simulink library "QuaternionLibrary"  (R2015a)
settings: Solver=ode45  StartTime=0.0  StopTime=10.0  RelTol=1e-3
libraries: VectorLibrary x2, ZeroProtectionLibrary x1
settings Model: Creator=Cam  LastModifiedBy=Cam

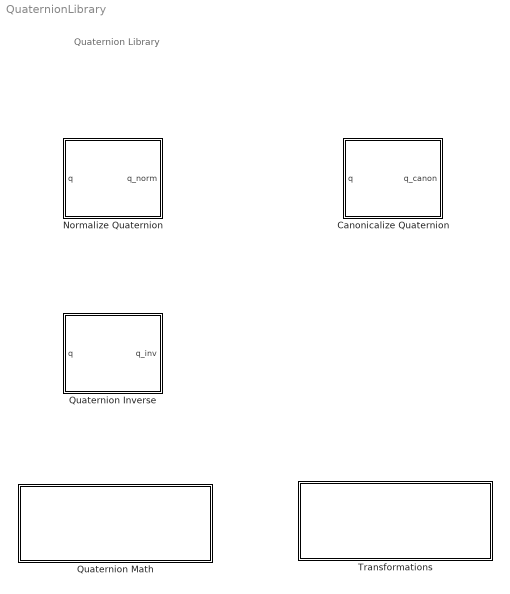
== system QuaternionLibrary ==
  note: Quaternion Library
  Canonicalize Quaternion : Subsystem  mask(Canonicalize Quaternion){}
      mask help: Returns the canonicalized form of the quaternion. This ensures that the angle is less than 180 degrees.
      mask Display: disp('Canonicalize\nQuaternion')
  Normalize Quaternion : Subsystem  mask(Normalize Quaternion){}
      mask help: Normalizes the given quaternion.
      mask Display: disp('Normalize\nQuaternion')
  Quaternion Inverse : Subsystem  mask(Quaternion Inverse){}
      mask help:
      | Returns the inverse of the given quaternion. That is, returns the quaternion that represents a rotation of the same angle, but about the negative of the axis.
      |
      | Exit condition:
      |  - The canonicalization status of the quaternion is preserved.
      mask Display: disp('Quaternion\nInverse')
  Quaternion Math : Subsystem
      mask Display: disp('Quaternion Math')
  Transformations : Subsystem
      mask Display: disp('Transformations')

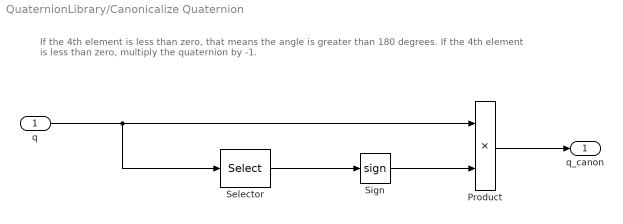
== system QuaternionLibrary/Canonicalize Quaternion ==
  note: If the 4th element is less than zero, that means the angle is greater than 180 degrees.
      | If the 4th element is less than zero, multiply the quaternion by -1.
  q : Inport
  Product : Product
  Selector : Selector  InputPortWidth=4  Indices=[4]
  Sign : Signum
  q_canon : Outport
  wires:
  q/1 -> Selector/1, Product/1
  Product/1 -> q_canon/1
  Sign/1 -> Product/2
  Selector/1 -> Sign/1

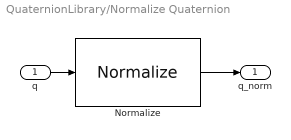
== system QuaternionLibrary/Normalize Quaternion ==
  q : Inport
  Normalize : VectorLibrary/Normalize
  q_norm : Outport
  wires:
  q/1 -> Normalize/1
  Normalize/1 -> q_norm/1

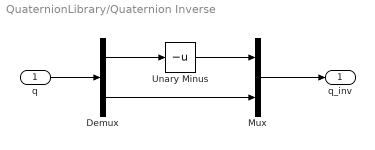
== system QuaternionLibrary/Quaternion Inverse ==
  q : Inport
  Demux : Demux  Outputs=2
  Mux : Mux  Inputs=2
  Unary Minus : UnaryMinus
  q_inv : Outport
  wires:
  Mux/1 -> q_inv/1
  q/1 -> Demux/1
  Demux/1 -> Unary Minus/1
  Unary Minus/1 -> Mux/1
  Demux/2 -> Mux/2

== system QuaternionLibrary/Quaternion Math ==
  note: Quaternion Math

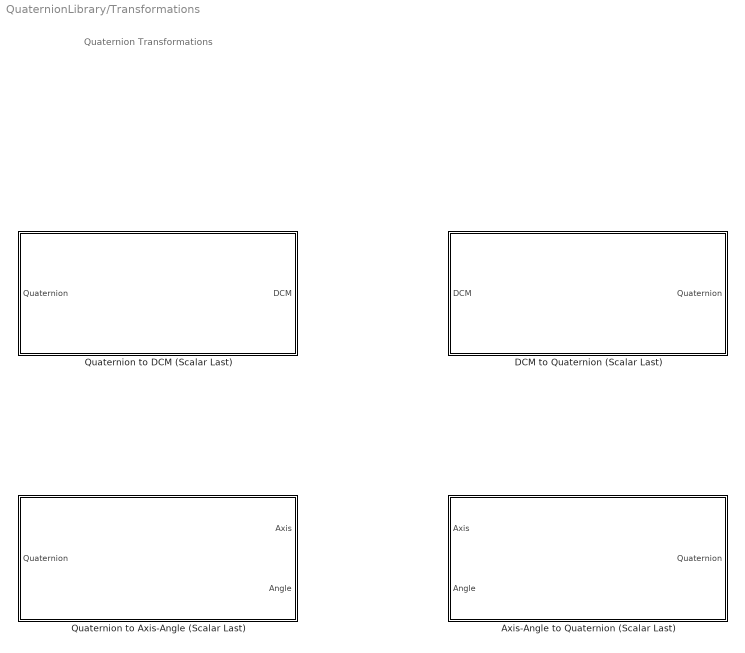
== system QuaternionLibrary/Transformations ==
  note: Quaternion Transformations
  Axis-Angle to Quaternion (Scalar Last) : Subsystem  mask(Axis-Angle to Quaternion){}
      mask help:
      | Returns the quaternion that represents a rotation of the given angle around the given axis.
      |
      | Entry condition:
      |  - Axis vector is normalized.
      mask Display:
      | port_label('input',1,'Axis')
      | port_label('input',2,'Angle')
      | port_label('output',1,'Quaternion')
      | disp('Axis-Angle \nto Quaternion\n')
      | color('red')
      | disp('\n\n(Scalar Last)')
  DCM to Quaternion (Scalar Last) : Subsystem  mask(DCM to Quaternion){}
      mask help:
      | This block transforms a DCM into a Quaternion.
      |
      | Entry condition:
      |  - Rows of DCM must be normalized.
      mask Display:
      | port_label('input',1,'DCM')
      | port_label('output',1,'Quaternion')
      | disp('Quaternion \nto DCM\n')
      | color('red')
      | disp('\n\n(Scalar Last)')
  Quaternion to Axis-Angle (Scalar Last) : Subsystem  mask(Quaternion to Axis-Angle){}
      mask help:
      | Returns the Euler axis and rotation angle about that axis that the quaternion represents.
      |
      | Entry Condition:
      |  - Quaternion is normalized.
      |
      | Exit condition:
      |  - Axis is normalized.
      |  - Canonicalization status is unchanged.
      mask Display:
      | port_label('input',1,'Quaternion')
      | port_label('output',1,'Axis')
      | port_label('output',2,'Angle')
      | disp('Quaternion \nto Axis-Angle\n')
      | color('red')
      | disp('\n\n(Scalar Last)')
  Quaternion to DCM (Scalar Last) : Subsystem  TreatAsAtomicUnit=on  mask(Quaternion to DCM){}
      mask help:
      | This block transforms a Quaternion into a Direction Cosine Matrix.
      |
      | Entry condition:
      |  - Quaternion must be normalized.
      mask Display:
      | port_label('input',1,'Quaternion')
      | port_label('output',1,'DCM')
      | disp('Quaternion \nto DCM\n')
      | color('red')
      | disp('\n\n(Scalar Last)')

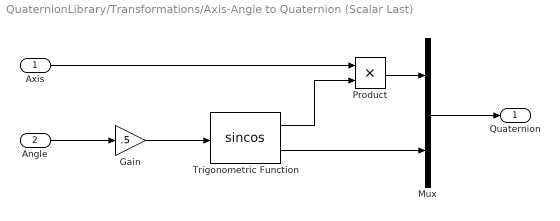
== system QuaternionLibrary/Transformations/Axis-Angle to Quaternion (Scalar Last) ==
  Axis : Inport
  Angle : Inport  Port=2
  Gain : Gain  Gain=.5
  Mux : Mux  Inputs=2
  Product : Product
  Trigonometric Function : Trigonometry  Operator=sincos
  Quaternion : Outport
  wires:
  Mux/1 -> Quaternion/1
  Angle/1 -> Gain/1
  Gain/1 -> Trigonometric Function/1
  Trigonometric Function/2 -> Mux/2
  Axis/1 -> Product/1
  Product/1 -> Mux/1
  Trigonometric Function/1 -> Product/2

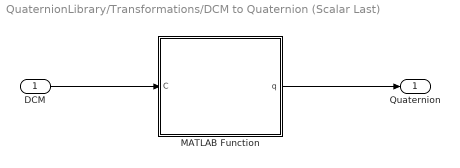
== system QuaternionLibrary/Transformations/DCM to Quaternion (Scalar Last) ==
  DCM : Inport
  MATLAB Function : MATLAB Function  TreatAsAtomicUnit=on
  Quaternion : Outport
  wires:
  DCM/1 -> MATLAB Function/1(C)
  MATLAB Function/1(q) -> Quaternion/1

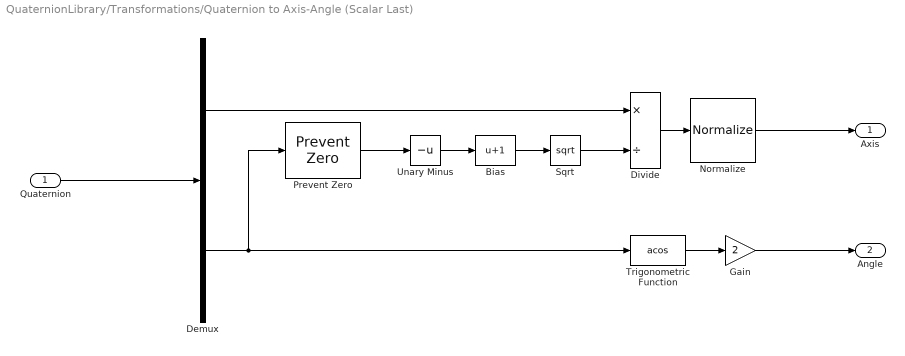
== system QuaternionLibrary/Transformations/Quaternion to Axis-Angle (Scalar Last) ==
  Quaternion : Inport
  Bias : Bias  Bias=1
  Demux : Demux  Outputs=[3 1]
  Divide : Product  Inputs=*/
  Gain : Gain  Gain=2
  Normalize : VectorLibrary/Normalize
  Prevent Zero : ZeroProtectionLibrary/Prevent Zero  thresh=0.0001
  Sqrt : Sqrt  SaturateOnIntegerOverflow=on
  Trigonometric Function : Trigonometry  Operator=acos
  Unary Minus : UnaryMinus
  Axis : Outport
  Angle : Outport  Port=2
  wires:
  Divide/1 -> Normalize/1
  Quaternion/1 -> Demux/1
  Demux/1 -> Divide/1
  Demux/2 -> Prevent Zero/1, Trigonometric Function/1
  Trigonometric Function/1 -> Gain/1
  Gain/1 -> Angle/1
  Unary Minus/1 -> Bias/1
  Bias/1 -> Sqrt/1
  Sqrt/1 -> Divide/2
  Prevent Zero/1 -> Unary Minus/1
  Normalize/1 -> Axis/1

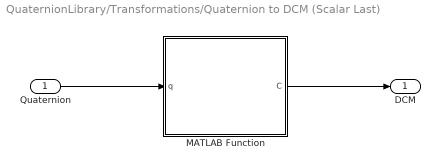
== system QuaternionLibrary/Transformations/Quaternion to DCM (Scalar Last) ==
  Quaternion : Inport
  MATLAB Function : MATLAB Function  TreatAsAtomicUnit=on
  DCM : Outport
  wires:
  Quaternion/1 -> MATLAB Function/1(q)
  MATLAB Function/1(C) -> DCM/1

== matlab function QuaternionLibrary/Transformations/DCM to Quaternion (Scalar Last)/MATLAB Function ==
  data: q output; C input
function q = DCM2Quat(C)
%#codegen

q4 = 1/2*sqrt(1+C(1,1)+C(2,2)+C(3,3));
q1 = 1/(4*q4)*(C(3,2)-C(2,3));
q2 = 1/(4*q4)*(C(1,3)-C(3,1));
q3 = 1/(4*q4)*(C(2,1)-C(1,2));

q = [q1 q2 q3 q4]';

== matlab function QuaternionLibrary/Transformations/Quaternion to DCM (Scalar Last)/MATLAB Function ==
  data: q input; C output
function C = Quat2DCM(q)
%#codegen

Q_cross = [  0      -q(3)    q(2)  ;
             q(3)   0       -q(1)  ;
            -q(2)    q(1)    0     ];


C = (q(4)^2-q(1:3)'*q(1:3))*eye(3) + 2*q(1:3)*q(1:3) + 2*q(4)*Q_cross;
